simulink model "temp"  (R2016b)
settings: Solver=VariableStepAuto  StartTime=0.0  StopTime=10.0  RelTol=1e-3
values from neighbouring files (symbols this model uses):
  fsw_params = init_fsw_params()    [momentum_unload_test_init.m]
libraries: momentum_dump_lib_test x1
settings Model: Creator=evich  LastModifiedBy=evich

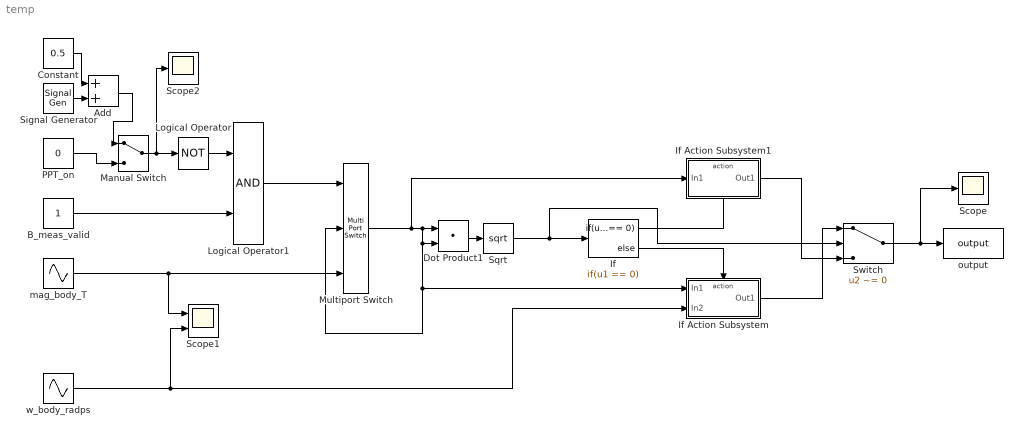
== system temp ==
  Add : Sum
  B_meas_valid : Constant
  Constant : Constant  Value=0.5
  Dot Product1 : DotProduct  InputSameDT=on  OutDataTypeStr=Inherit: Inherit via internal rule
  If : If  IfExpression=u1 == 0
  If Action Subsystem : Subsystem  TreatAsAtomicUnit=on
  If Action Subsystem1 : Subsystem  TreatAsAtomicUnit=on
  Logical Operator : Logic  Operator=NOT  AllPortsSameDT=off  OutDataTypeStr=boolean
  Logical Operator1 : Logic  AllPortsSameDT=off  OutDataTypeStr=boolean
  Manual Switch : ManualSwitch
  Multiport Switch : MultiPortSwitch  DataPortOrder=Zero-based contiguous  Inputs=2
  PPT_on : Constant  Value=0
  Scope : Scope
  Scope1 : Scope  NumInputPorts=2
  Scope2 : Scope
  Signal Generator : SignalGenerator  WaveForm=square  Amplitude=0.5  Frequency=1.5  Units=rad/sec
  Sqrt : Sqrt  SaturateOnIntegerOverflow=on
  Switch : Switch  Criteria=u2 ~= 0
  mag_body_T : Sin  Amplitude=[2 1 7]'  Bias=[2 1 7]'  Frequency=[1 2 1]'  Phase=[0 0 pi()/4]'  SampleTime=0  VectorParams1D=off
  output : ToWorkspace  VariableName=output  SaveFormat=Structure  SampleTime=-1
  w_body_radps : Sin  Amplitude=[1 4 2]'  Bias=[1 4 2]'  Frequency=[1 2 5]'  Phase=[0 pi()/2 0]'  SampleTime=0  VectorParams1D=off
  wires:
  Logical Operator1/1 -> Multiport Switch/1
  Logical Operator/1 -> Logical Operator1/1
  B_meas_valid/1 -> Logical Operator1/2
  mag_body_T/1 -> Multiport Switch/3, Scope1/1
  Multiport Switch/1 -> If Action Subsystem1/1(In1), Dot Product1/2, Multiport Switch/2, If Action Subsystem/1(In1), Dot Product1/1
  w_body_radps/1 -> If Action Subsystem/2(In2), Scope1/2
  Switch/1 -> Scope/1, output/1
  Dot Product1/1 -> Sqrt/1
  Sqrt/1 -> Switch/2, If/1
  If/2 -> If Action Subsystem/Action
  If/1 -> If Action Subsystem1/Action
  If Action Subsystem1/1(Out1) -> Switch/3
  If Action Subsystem/1(Out1) -> Switch/1
  Manual Switch/1 -> Scope2/1, Logical Operator/1
  PPT_on/1 -> Manual Switch/2
  Constant/1 -> Add/1
  Signal Generator/1 -> Add/2
  Add/1 -> Manual Switch/1

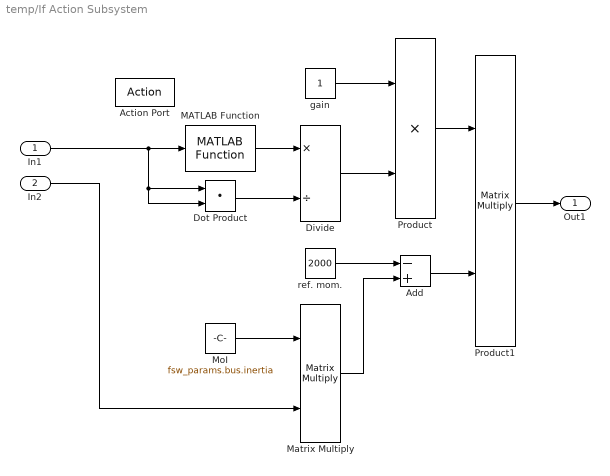
== system temp/If Action Subsystem ==
  In1 : Inport
  In2 : Inport  Port=2
  Action Port : ActionPort  ActionType=else
  Add : Sum  Inputs=-+
  Divide : Product  Inputs=*/
  Dot Product : DotProduct  InputSameDT=on  OutDataTypeStr=Inherit: Inherit via internal rule
  MATLAB Function : momentum_dump_lib_test/Momentum unloading/MATLAB Function
  Matrix Multiply : Product  Inputs=**  Multiplication=Matrix(*)
  MoI : Constant  Value=fsw_params.bus.inertia
  Product : Product  Inputs=**
  Product1 : Product  Inputs=**  Multiplication=Matrix(*)
  gain : Constant
  ref. mom. : Constant  Value=2000
  Out1 : Outport
  wires:
  Divide/1 -> Product/2
  Dot Product/1 -> Divide/2
  gain/1 -> Product/1
  ref. mom./1 -> Add/1
  Matrix Multiply/1 -> Add/2
  Product/1 -> Product1/1
  Add/1 -> Product1/2
  MATLAB Function/1 -> Divide/1
  MoI/1 -> Matrix Multiply/1
  In1/1 -> Dot Product/2, Dot Product/1, MATLAB Function/1
  In2/1 -> Matrix Multiply/2
  Product1/1 -> Out1/1

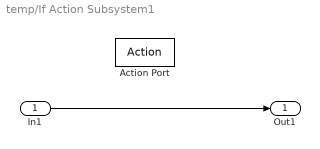
== system temp/If Action Subsystem1 ==
  In1 : Inport
  Action Port : ActionPort  ActionType=then
  Out1 : Outport
  wires:
  In1/1 -> Out1/1
